simulink model "LR_4_var2"  (R2020b)
settings: Solver=FixedStepAuto  StartTime=0.0  StopTime=60  FixedStep=1e-4  RelTol=1e-3
settings Model: Creator=SIA  LastModifiedBy=SIA

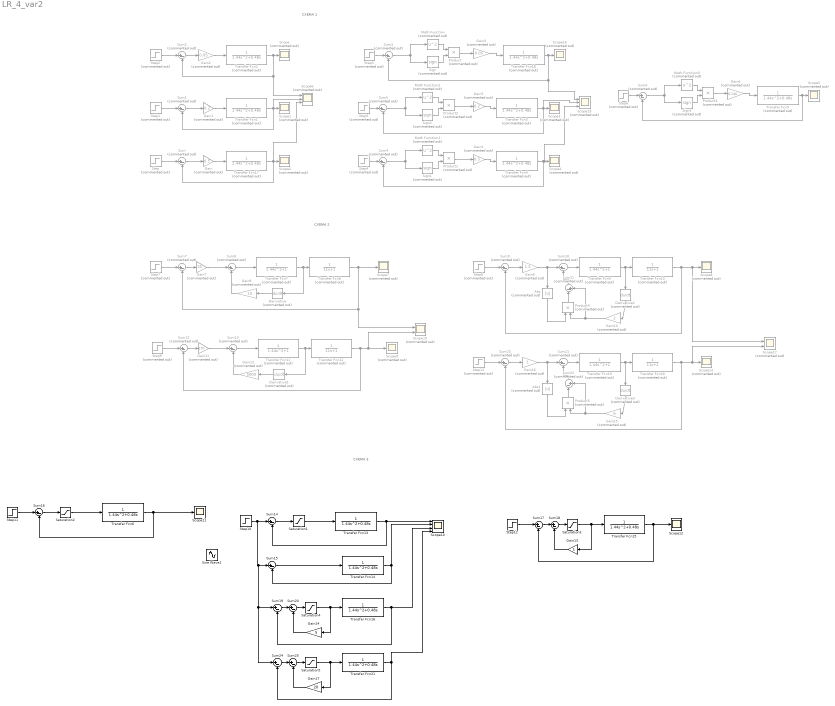
== system LR_4_var2 ==
  note: СХЕМА 1
  note: СХЕМА 2
  note: СХЕМА 3
  Abs : Abs  Commented=on
  Abs1 : Abs  Commented=on
  Derivative{,1..3} (4 alike) : Derivative  Commented=on
  Gain : Gain  Commented=on  Gain=0.5
  Gain1 : Gain  Commented=on  Gain=0.2
  Gain10 : Gain  Commented=on  Gain=2
  Gain11 : Gain  Commented=on  Gain=170
  Gain12 : Gain  Commented=on  Gain=5000
  Gain13 : Gain
  Gain14 : Gain  Gain=5
  Gain15 : Gain  Commented=on  Gain=6
  Gain16 : Gain  Commented=on
  Gain17 : Gain  Gain=20
  Gain2 : Gain  Commented=on  Gain=0.05
  Gain3 : Gain  Commented=on  Gain=0.05
  Gain4 : Gain  Commented=on  Gain=0.5
  Gain5 : Gain  Commented=on  Gain=0.2
  Gain6 : Gain  Commented=on  Gain=0.136
  Gain7 : Gain  Commented=on  Gain=35
  Gain8 : Gain  Commented=on  Gain=10
  Gain9 : Gain  Commented=on  Gain=1.5
  Math Function{,1..3} (4 alike) : Math  Commented=on  Operator=square  SaturateOnIntegerOverflow=on
  Product{,1..5} (6 alike) : Product  Commented=on
  Saturation{1..5} (5 alike) : Saturate
  Scope{,1..5,7..9,14,16} (11 alike) : Scope  Commented=on
  Scope10 : Scope  NumInputPorts=4
  Scope11 : Scope
  Scope12 : Scope
  Scope13 : Scope  Commented=on  NumInputPorts=3
  Scope15 : Scope  Commented=on  NumInputPorts=2
  Scope17 : Scope  Commented=on  NumInputPorts=2
  Scope6 : Scope  Commented=on  NumInputPorts=3
  Sign{,1..3} (4 alike) : Signum  Commented=on
  Sine Wave1 : Sin  SampleTime=0
  Step{,1..9,13} (11 alike) : Step  Commented=on  Time=0  SampleTime=0
  Step10 : Step  Time=0  After=10  SampleTime=0
  Step11 : Step  Time=0  After=10  SampleTime=0
  Step12 : Step  Time=0  After=10  SampleTime=0
  Sum{,1..10,12..13,21,23} (15 alike) : Sum  Commented=on  Inputs=|+-
  Sum11 : Sum  Commented=on  Inputs=|-+
  Sum{14..20,24..25} (9 alike) : Sum  Inputs=|+-
  Sum22 : Sum  Commented=on  Inputs=|-+
  Transfer Fcn{1..5,17..18} (7 alike) : TransferFcn  Commented=on  Denominator=[1.44 0.48 0]
  Transfer Fcn{8,10,12,20} (4 alike) : TransferFcn  Commented=on  Denominator=[11 1]
  Transfer Fcn{7,9,11,19} (4 alike) : TransferFcn  Commented=on  Denominator=[1.44 0 1]
  Transfer Fcn{6,13..16,21} (6 alike) : TransferFcn  Denominator=[1.44 0.48 0]
  wires:
  Step/1 -> Sum/1
  Sum/1 -> Gain/1
  Gain/1 -> Transfer Fcn17/1
  Transfer Fcn17/1 -> Scope6/3, Scope2/1, Sum/2
  Gain1/1 -> Transfer Fcn1/1
  Sum1/1 -> Gain1/1
  Transfer Fcn1/1 -> Scope6/2, Scope1/1, Sum1/2
  Step1/1 -> Sum1/1
  Gain2/1 -> Transfer Fcn2/1
  Sum2/1 -> Gain2/1
  Transfer Fcn2/1 -> Scope/1, Scope6/1, Sum2/2
  Step2/1 -> Sum2/1
  Step3/1 -> Sum3/1
  Sum3/1 -> Sign/1, Math Function/1
  Transfer Fcn18/1 -> Scope16/1, Scope13/1, Sum3/2
  Math Function/1 -> Product/1
  Sign/1 -> Product/2
  Gain3/1 -> Transfer Fcn18/1
  Product/1 -> Gain3/1
  Math Function1/1 -> Product1/1
  Product1/1 -> Gain4/1
  Sum4/1 -> Sign1/1, Math Function1/1
  Gain4/1 -> Transfer Fcn4/1
  Step4/1 -> Sum4/1
  Sign1/1 -> Product1/2
  Transfer Fcn4/1 -> Scope13/3, Scope4/1, Sum4/2
  Math Function2/1 -> Product2/1
  Product2/1 -> Gain5/1
  Sum5/1 -> Sign2/1, Math Function2/1
  Gain5/1 -> Transfer Fcn3/1
  Step5/1 -> Sum5/1
  Sign2/1 -> Product2/2
  Transfer Fcn3/1 -> Scope13/2, Scope3/1, Sum5/2
  Math Function3/1 -> Product3/1
  Product3/1 -> Gain6/1
  Sum6/1 -> Sign3/1, Math Function3/1
  Gain6/1 -> Transfer Fcn5/1
  Step6/1 -> Sum6/1
  Sign3/1 -> Product3/2
  Transfer Fcn5/1 -> Scope5/1, Sum6/2
  Transfer Fcn7/1 -> Derivative/1, Transfer Fcn8/1
  Sum7/1 -> Gain7/1
  Step7/1 -> Sum7/1
  Transfer Fcn8/1 -> Scope15/1, Sum7/2, Scope7/1
  Gain7/1 -> Sum8/1
  Sum8/1 -> Transfer Fcn7/1
  Gain8/1 -> Sum8/2
  Gain9/1 -> Abs/1, Sum10/1
  Transfer Fcn9/1 -> Transfer Fcn10/1, Derivative2/1
  Sum9/1 -> Gain9/1
  Step8/1 -> Sum9/1
  Sum10/1 -> Transfer Fcn9/1
  Product4/1 -> Sum11/1
  Gain10/1 -> Sum11/2, Product4/2
  Derivative/1 -> Gain8/1
  Derivative2/1 -> Gain10/1
  Transfer Fcn13/1 -> Scope10/1, Sum14/2
  Sum14/1 -> Saturation1/1
  Saturation1/1 -> Transfer Fcn13/1
  Sum15/1 -> Transfer Fcn14/1
  Transfer Fcn14/1 -> Scope10/2, Sum15/2
  Saturation2/1 -> Transfer Fcn6/1
  Step11/1 -> Sum16/1
  Transfer Fcn6/1 -> Scope11/1, Sum16/2
  Sum16/1 -> Saturation2/1
  Transfer Fcn15/1 -> Sum17/2, Scope12/1
  Saturation3/1 -> Transfer Fcn15/1, Gain13/1
  Step12/1 -> Sum17/1
  Sum17/1 -> Sum18/1
  Sum18/1 -> Saturation3/1
  Gain13/1 -> Sum18/2
  Sum20/1 -> Saturation4/1
  Sum19/1 -> Sum20/1
  Saturation4/1 -> Transfer Fcn16/1, Gain14/1
  Gain14/1 -> Sum20/2
  Transfer Fcn16/1 -> Scope10/3, Sum19/2
  Sum11/1 -> Sum10/2
  Abs/1 -> Product4/1
  Sum12/1 -> Gain11/1
  Sum13/1 -> Transfer Fcn11/1
  Step9/1 -> Sum12/1
  Derivative1/1 -> Gain12/1
  Gain12/1 -> Sum13/2
  Transfer Fcn12/1 -> Sum12/2, Scope9/1, Scope15/2
  Transfer Fcn11/1 -> Transfer Fcn12/1, Derivative1/1
  Gain11/1 -> Sum13/1
  Transfer Fcn20/1 -> Scope17/2, Scope14/1, Sum23/2
  Step13/1 -> Sum23/1
  Product5/1 -> Sum22/1
  Sum23/1 -> Gain16/1
  Gain16/1 -> Abs1/1, Sum21/1
  Gain15/1 -> Sum22/2, Product5/2
  Abs1/1 -> Product5/1
  Transfer Fcn19/1 -> Transfer Fcn20/1, Derivative3/1
  Sum22/1 -> Sum21/2
  Sum21/1 -> Transfer Fcn19/1
  Derivative3/1 -> Gain15/1
  Transfer Fcn10/1 -> Scope17/1, Scope8/1, Sum9/2
  Gain17/1 -> Sum25/2
  Saturation5/1 -> Transfer Fcn21/1, Gain17/1
  Sum24/1 -> Sum25/1
  Step10/1 -> Sum24/1, Sum19/1, Sum15/1, Sum14/1
  Transfer Fcn21/1 -> Scope10/4, Sum24/2
  Sum25/1 -> Saturation5/1
